simulink model "twodof_evaluation"  (R2019a)
settings: Solver=VariableStepAuto  StartTime=0.0  StopTime=10.0  RelTol=1e-3
libraries: fl_lib x7, nesl_utility x5, eeGeneralControl x2
settings Model: Creator=Owen Heaney  LastModifiedBy=Owen Heaney
settings SimscapeCC: SimscapeNormalizeSystem=off

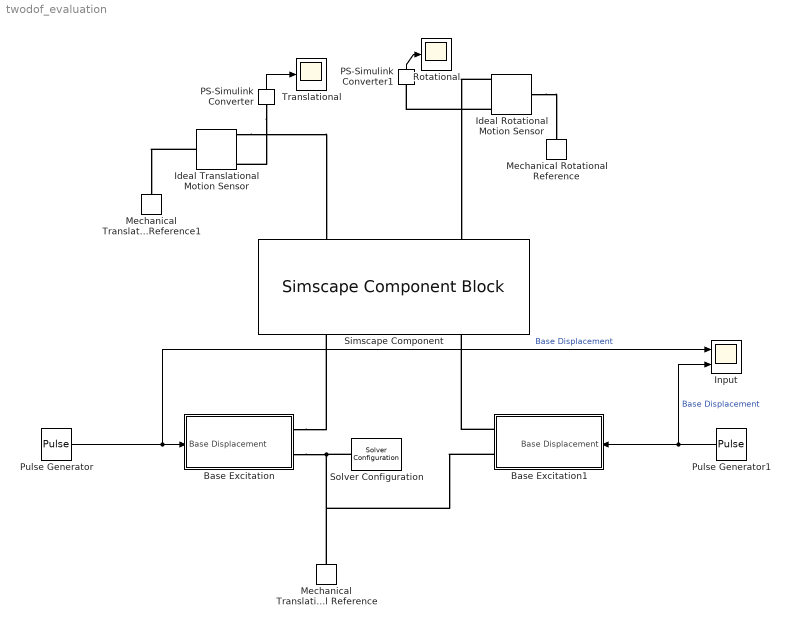
== system twodof_evaluation ==
  Base Excitation : Subsystem
  Base Excitation1 : Subsystem
  Ideal Rotational Motion Sensor : fl_lib/Mechanical/Mechanical Sensors/Ideal Rotational Motion Sensor  offset=0 rad
  Ideal Translational Motion Sensor : fl_lib/Mechanical/Mechanical Sensors/Ideal Translational Motion Sensor  offset=0 m
  Input : Scope  NumInputPorts=2
  Mechanical Rotational Reference : fl_lib/Mechanical/Rotational Elements/Mechanical Rotational Reference
  Mechanical Translational Reference : fl_lib/Mechanical/Translational Elements/Mechanical Translational Reference
  Mechanical Translational Reference1 : fl_lib/Mechanical/Translational Elements/Mechanical Translational Reference
  PS-Simulink Converter : nesl_utility/PS-Simulink Converter  PhysicalDomain=network_engine_domain  SubClassName=ps_output  LeftPortType=input  RightPortType=output  PseudoPeriodic=off  Frequencies=[]  Unit=1  AffineConversion=off
  PS-Simulink Converter1 : nesl_utility/PS-Simulink Converter  PhysicalDomain=network_engine_domain  SubClassName=ps_output  LeftPortType=input  RightPortType=output  PseudoPeriodic=off  Frequencies=[]  Unit=1  AffineConversion=off
  Pulse Generator : DiscretePulseGenerator  PulseType=Time based  Period=10  PulseWidth=50  PhaseDelay=6
  Pulse Generator1 : DiscretePulseGenerator  PulseType=Time based  Period=10  PulseWidth=50
  Rotational : Scope
  Simscape Component : SimscapeComponentBlock  SourceFile=TwoDoFChassis  ComponentPath=TwoDoFChassis  ComponentVariants=TwoDoFChassis  ComponentVariantNames=TwoDoFChassis  ClassName=TwoDoFChassis  SchemaVersion=1  a=2 m  b=1 m  M_specify=off  M_priority=None  M=0 N*m  M_nominal_specify=off  M_nominal_unit=N*m  M_nominal_value=1  F_specify=off  F_priority=None  F=0 N  F_nominal_specify=off  F_nominal_unit=N  F_nominal_value=1  F_f_specify=off  F_f_priority=None  F_f=0 N  F_f_nominal_specify=off  F_f_nominal_unit=N  F_f_nominal_value=1  F_r_specify=off  F_r_priority=None  F_r=0 N  F_r_nominal_specify=off  F_r_nominal_unit=N  F_r_nominal_value=1
      settings: CopyFcn=simscape.engine.sli.internal.componentblockcallback(gcbh,'COPY')  PreCopyFcn=simscape.engine.sli.internal.componentblockcallback(gcbh,'PRECOPY')  PreDeleteFcn=simscape.engine.sli.internal.componentblockcallback(gcbh,'PREDELETE')
      mask Type: TwoDoFChassis
  Solver Configuration : nesl_utility/Solver Configuration  PhysicalDomain=network_engine_domain  SubClassName=solver  LeftPortType=input  RightPortType=generic  Tones=[]  Harmonics=[]  SimulateNoise=off  Profile=off  UseLocalSampling=off  EnableSwitchedLinearOptims=on  FrequencyDomain=off  UseCCode=off  RelTol=0.001  AbsTol=1e-06  MinStep=1e-09  ToWorkspace=off  RevertToSquareIcSolve=off  NumHomotopyIterations=100  PhasorMode=off  PhasorModeNumHarmonics=1  DoDC=on  ResidualTolerance=1e-15  UseLocalSolver=off  LocalSolverChoice=NE_BACKWARD_EULER_ADVANCER  LocalSolverSampleTime=0.001  DoFixedCost=off  MaxNonlinIter=3  MaxModeIter=2  LinearAlgebra=auto  EquationFormulation=NE_TIME_EF  DelaysMemoryBudget=1024  AutomaticFiltering=on  FilteringTimeConstant=0.001  PartitionStorageMethod=AS_NEEDED  PartitionMemoryBudget=1024  PartitionMethod=ROBUST
  Translational : Scope
  wires:
  Pulse Generator/1 -> Input/1, Base Excitation/1(Base Displacement)  "Base Displacement"
  Pulse Generator1/1 -> Input/2, Base Excitation1/1(Base Displacement)  "Base Displacement"
  PS-Simulink Converter/1 -> Translational/1
  PS-Simulink Converter1/1 -> Rotational/1
  connections:
  Base Excitation/RConn2 -- Base Excitation1/RConn2 -- Mechanical Translational Reference/LConn1 -- Solver Configuration/RConn1
  Base Excitation1/RConn1 -- Simscape Component/LConn2
  Ideal Translational Motion Sensor/LConn1 -- Mechanical Translational Reference1/LConn1
  Ideal Translational Motion Sensor/RConn1 -- Simscape Component/RConn1
  PS-Simulink Converter/LConn1 -- Ideal Translational Motion Sensor/RConn3
  Base Excitation/RConn1 -- Simscape Component/LConn1
  Ideal Rotational Motion Sensor/LConn1 -- Mechanical Rotational Reference/LConn1
  Ideal Rotational Motion Sensor/RConn1 -- Simscape Component/RConn2
  Ideal Rotational Motion Sensor/RConn3 -- PS-Simulink Converter1/LConn1

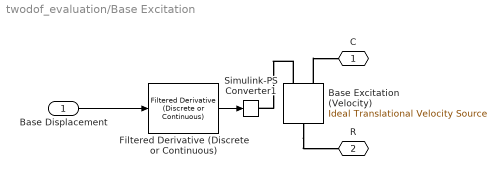
== system twodof_evaluation/Base Excitation ==
  Base Displacement : Inport
  Base Excitation (Velocity) : fl_lib/Mechanical/Mechanical Sources/Ideal Translational Velocity Source
  Filtered Derivative (Discrete or Continuous) : eeGeneralControl/Filtered Derivative (Discrete or Continuous)  K=1  T=0.0001  B=inf  A=-inf  minRatio=10  Ts=0
      settings: SourceProductName=Simscape Electrical  SourceProductBaseCode=PS
  Simulink-PS Converter1 : nesl_utility/Simulink-PS Converter  PhysicalDomain=network_engine_domain  SubClassName=ps_input  LeftPortType=input  RightPortType=output  PseudoPeriodic=off  Frequencies=[]  NoiseDistribution=none  NoiseParameters=[]  Unit=mm/s  AffineConversion=off  FilteringAndDerivatives=filter  SimscapeFilterOrder=1  InputFilterTimeConstant=0.001  UdotUserProvided=0
  C : PMIOPort  Side=Right
  R : PMIOPort  Port=2  Side=Right
  wires:
  Base Displacement/1 -> Filtered Derivative (Discrete or Continuous)/1
  Filtered Derivative (Discrete or Continuous)/1 -> Simulink-PS Converter1/1
  connections:
  Base Excitation (Velocity)/RConn1 -- Simulink-PS Converter1/RConn1
  Base Excitation (Velocity)/RConn2 -- C/RConn1
  Base Excitation (Velocity)/LConn1 -- R/RConn1

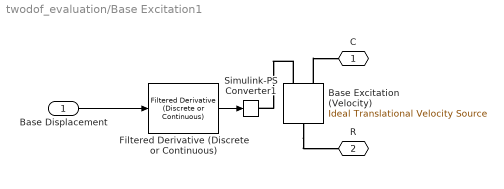
== system twodof_evaluation/Base Excitation1 ==
  Base Displacement : Inport
  Base Excitation (Velocity) : fl_lib/Mechanical/Mechanical Sources/Ideal Translational Velocity Source
  Filtered Derivative (Discrete or Continuous) : eeGeneralControl/Filtered Derivative (Discrete or Continuous)  K=1  T=0.0001  B=inf  A=-inf  minRatio=10  Ts=0
      settings: SourceProductName=Simscape Electrical  SourceProductBaseCode=PS
  Simulink-PS Converter1 : nesl_utility/Simulink-PS Converter  PhysicalDomain=network_engine_domain  SubClassName=ps_input  LeftPortType=input  RightPortType=output  PseudoPeriodic=off  Frequencies=[]  NoiseDistribution=none  NoiseParameters=[]  Unit=mm/s  AffineConversion=off  FilteringAndDerivatives=filter  SimscapeFilterOrder=1  InputFilterTimeConstant=0.001  UdotUserProvided=0
  C : PMIOPort  Side=Right
  R : PMIOPort  Port=2  Side=Right
  wires:
  Filtered Derivative (Discrete or Continuous)/1 -> Simulink-PS Converter1/1
  Base Displacement/1 -> Filtered Derivative (Discrete or Continuous)/1
  connections:
  Base Excitation (Velocity)/LConn1 -- R/RConn1
  Base Excitation (Velocity)/RConn2 -- C/RConn1
  Base Excitation (Velocity)/RConn1 -- Simulink-PS Converter1/RConn1
